simulink model "MTDC_MODEL"  (R2021a)
settings: Solver=ode1  StartTime=0.0  StopTime=3  FixedStep=2e-5  MaxStep=1e-5  RelTol=1e-5  EnableMultiTasking=on
InitFcn:
  | tau_iac=ts_G_iac/4;                                         %Current loop speed
  | wAC=1/tau_iac;                                              %Frequency
  | L1AC=wAC/s;                                                 %Open loop IMC (L) transfer function to obtain a first order after closing the loop
  | Kp_AC=wAC*(Lg_1+La_1/2);                                    %Proportional constant of the controller
  | Ki_AC=wAC*(Rg_1+Ra_1/2);                                    %Integral constant of the controller
  | C_IMC_AC=(Kp_AC*s+Ki_AC)/s;                                 %IMC designed PI controller transfer function
  | TAC=minreal((C_IMC_AC)*G_iac/(1+(C_IMC_AC)*G_iac));         %Closed loop transfer function
  | 
  | tau_Pac=ts_G_P/4;
  | D = TAC*U_ll1;
  | [C_pi,info] = pidtune(D,'PI',1/tau_Pac);
  | Ki_P = C_pi.Ki;
  | 
  | tau_Qac=ts_G_Q/4;
  | [C_piq,info] = pidtune(D,'PI',1/tau_Qac);
  | Ki_Q = C_piq.Ki;
  | 
  | 
  | tau_isum=ts_G_isum/4;                                        %Current loop speed
  | wsum=1/tau_isum;                                             %Frequency
  | L1AC=wsum/s;                                                 %Open loop IMC (L) transfer function to obtain a first order after closing the loop
  | Kp_sum=wsum*(2*La_1);                                        %Proportional constant of the controller
  | Ki_sum=wsum*(2*Ra_1);                                        %Integral constant of the controller
  | C_IMC_sum=(Kp_sum*s+Ki_sum)/s;                               %IMC designed PI controller transfer function
  | 
  | Kp_sum_PR = wc*(2*La_1);
  | Ki_sum_PR = wc*(2*Ra_1);
  | PR = (Kp_sum_PR*s^2 + 2*wc*(Kp_sum_PR+Ki_sum_PR)*s +Kp_sum_PR*w0^2)/(s^2+2*wc*s+w0^2);
  | 
  | 
  | %Energy reference for a converter arm (sum of all the submodule energies)
  | ArmEnergyRef=1/2*Carm*ArmVoltageRef^2;                      %Energy reference for a converter leg
  | LegEnergy=ArmEnergyRef*2;                                   %References for the controllers (DC side)
  | TotalEnergyRef=ArmEnergyRef*6;                              %Reference of the total energy of the converter
  | EnergyDiffabRef=0;                                          %Reference for the energy difference between legs a and b
  | EnergyDiffacRef=0;                                          %Reference for the energy difference between legs b and c
  | 
  | %References for the controllers (AC side)
  | EnergyDiffUpLowRefa=0;                                      %Reference for the energy difference upper and lower arms of phase a
  | EnergyDiffUpLowRefb=0;                                      %Reference for the energy difference upper and lower arms of phase b
  | EnergyDiffUpLowRefc=0;                                      %Reference for the energy difference upper and lower arms of phase c
  |                                                             %Controller design
  | Kpenergy=50;                                                %Proportional gain
  | Kienergy=20;                                                %Integral gain
  | 
  | Kpenergyt=50;                                               %Proportional gain
  | Kienergyt=20;                                               %Integral gain
  | 
  | Q=3;
  | wn=50*2*pi;                                                 %Frequency to eliminate 50 Hz
  | N_50 = tf([1 0 wn^2],[1 2*wn/Q wn^2]);                       %Notch filter 1 design
  | wn=100*2*pi;                                                %Frequency to eliminate 100 Hz
  | N_100 = tf([1 0 wn^2],[1 2*wn/Q wn^2]);                      %Notch filter 2 design
  | Notch=N_50*N_100;                                            %Combination of both notch filters
  | 
  | Ibasedc1= 1000e6/640e3;                 %Nominal current peak DC
  | IsaturationinnerDC1=1.1*Ibasedc1/3;  %Saturation of the DC inner current
  | IsaturationinnerAC1=0.45*Ibasedc1/3; %0.45  %Saturation of the inner current (why edu used 10% - FYI I changed it to 45%)
  | 
  | 
  | ... (+30 lines)
values from neighbouring files (symbols this model uses):
  ArmVoltageRef = 640e3    (= 640000)    [MMC_PARAMETERS.m]
  Cap = 9.5e-3    (= 0.0095)    [MMC_PARAMETERS.m]
  Carm = Cap/N    (= 2.375e-05)    [MMC_PARAMETERS.m]
  f_grid = 50    [MMC_PARAMETERS.m]
  La_1 = 0.15*Zbase_1/2/pi/50    (= 0.0488923985178)    [MMC_PARAMETERS.m]
  Lg_1 = 0.18*Zbase_1/2/pi/50    (= 0.0586708782214)    [MMC_PARAMETERS.m]
  N = 400    [MMC_PARAMETERS.m]
  Ra_1 = 0.01*Zbase_1    (= 1.024)    [MMC_PARAMETERS.m]
  Rg_1 = 0.005*Zbase_1    (= 0.512)    [MMC_PARAMETERS.m]
  S_1 = 1000e6    (= 1000000000)    [MMC_PARAMETERS.m]
  U_ll1 = 320e3    (= 320000)    [MMC_PARAMETERS.m]
  Vdc = 640e3    (= 640000)    [MMC_PARAMETERS.m]
  Vpeak_d1 = U_pnpeak1    [MMC_PARAMETERS.m]
  w0 = 2*pi*50    (= 314.159265359)    [MMC_PARAMETERS.m]
undefined symbols (not defined in the file or in its folder): Kp_Pac, lenght
libraries: spsSeriesRLCBranchLib x80, spsCurrentMeasurementLib x64, spsControlledVoltageSourceLib x36, pid_lib x32, spsVoltageMeasurementLib x32, spsControlledCurrentSourceLib x24, spsParallelRLCBranchLib x20, spsGroundLib x10, powerlib_extras x4, spsDCVoltageSourceLib x4, spspowerguiLib x1
(part 7 of 9)

== system MTDC_MODEL/GRID4+MMC4/Equivalent arm lower-a2 ==
  note: Power_lb
  vlb : Inport
  Controlled Current Source : spsControlledCurrentSourceLib/Controlled Current Source  Initialize=on  Source_Type=AC  Amplitude=0  Phase=0  Frequency=0  Measurements=None
  Controlled Voltage Source7 : spsControlledVoltageSourceLib/Controlled Voltage Source  Initialize=on  Source_Type=AC  Amplitude=Vdc/2  Phase=0  Frequency=0  Measurements=None
  Current Measurement4 : spsCurrentMeasurementLib/Current Measurement  PhasorSimulation=off  OutputType=Complex  PSBequivalent=0
  Divide1 : Product  Inputs=**
  Divide2 : Product  Inputs=*/
  Filtered Lower arm B instananeous power1 : Scope
  Gain : Gain  Gain=1e6
  Lower arm B instananeous power : Scope
  Series RLC Branch2 : spsSeriesRLCBranchLib/Series RLC Branch  LConnTagsString=__new0  RConnTagsString=__new0  BranchType=C  Resistance=Ra_1  Inductance=La_1  SetiL0=on  InitialCurrent=0  Capacitance=Cap/N  Setx0=on  InitialVoltage=640e3  Measurements=None
  Transfer Fcn : TransferFcn  Denominator=[1 1]
  Voltage Measurement : spsVoltageMeasurementLib/Voltage Measurement  PhasorSimulation=off  OutputType=Complex  PSBequivalent=0
  Conn1 : PMIOPort  Side=Right
  Conn2 : PMIOPort  Port=2  Side=Left
  v_sum_lb : Outport
  wires:
  Gain/1 -> Filtered Lower arm B instananeous power1/1
  Transfer Fcn/1 -> Gain/1
  Current Measurement4/1 -> Divide1/2  "ilb"
  Divide1/1 -> Divide2/1, Transfer Fcn/1, Lower arm B instananeous power/1
  Divide2/1 -> Controlled Current Source/1
  Voltage Measurement/1 -> Divide2/2, v_sum_lb/1
  vlb/1 -> Controlled Voltage Source7/1, Divide1/1  "vlb"
  connections:
  Conn2/RConn1 -- Current Measurement4/RConn1
  Current Measurement4/LConn1 -- Controlled Voltage Source7/LConn1
  Voltage Measurement/LConn2 -- Series RLC Branch2/RConn1 -- Controlled Current Source/LConn1
  Controlled Current Source/RConn1 -- Series RLC Branch2/LConn1 -- Voltage Measurement/LConn1
  Controlled Voltage Source7/RConn1 -- Conn1/RConn1

== system MTDC_MODEL/GRID4+MMC4/Equivalent arm lower-a3 ==
  note: Power_lc
  vlc : Inport
  Controlled Current Source : spsControlledCurrentSourceLib/Controlled Current Source  Initialize=on  Source_Type=AC  Amplitude=0  Phase=0  Frequency=0  Measurements=None
  Controlled Voltage Source7 : spsControlledVoltageSourceLib/Controlled Voltage Source  Initialize=on  Source_Type=AC  Amplitude=Vdc/2  Phase=0  Frequency=0  Measurements=None
  Current Measurement4 : spsCurrentMeasurementLib/Current Measurement  PhasorSimulation=off  OutputType=Complex  PSBequivalent=0
  Divide1 : Product  Inputs=**
  Divide2 : Product  Inputs=*/
  Filtered Lower arm A instananeous power1 : Scope
  Gain : Gain  Gain=1e6
  Lower arm A instananeous power : Scope
  Series RLC Branch2 : spsSeriesRLCBranchLib/Series RLC Branch  LConnTagsString=__new0  RConnTagsString=__new0  BranchType=C  Resistance=Ra_1  Inductance=La_1  SetiL0=on  InitialCurrent=0  Capacitance=Cap/N  Setx0=on  InitialVoltage=640e3  Measurements=None
  Transfer Fcn : TransferFcn  Denominator=[1 1]
  Voltage Measurement : spsVoltageMeasurementLib/Voltage Measurement  PhasorSimulation=off  OutputType=Complex  PSBequivalent=0
  Conn1 : PMIOPort  Side=Right
  Conn2 : PMIOPort  Port=2  Side=Left
  v_sum_lc : Outport
  wires:
  vlc/1 -> Divide1/1, Controlled Voltage Source7/1  "vla"
  Voltage Measurement/1 -> v_sum_lc/1, Divide2/2
  Divide2/1 -> Controlled Current Source/1
  Divide1/1 -> Lower arm A instananeous power/1, Transfer Fcn/1, Divide2/1
  Current Measurement4/1 -> Divide1/2  "ila"
  Transfer Fcn/1 -> Gain/1
  Gain/1 -> Filtered Lower arm A instananeous power1/1
  connections:
  Controlled Voltage Source7/RConn1 -- Conn1/RConn1
  Voltage Measurement/LConn1 -- Series RLC Branch2/LConn1 -- Controlled Current Source/RConn1
  Controlled Current Source/LConn1 -- Series RLC Branch2/RConn1 -- Voltage Measurement/LConn2
  Current Measurement4/LConn1 -- Controlled Voltage Source7/LConn1
  Conn2/RConn1 -- Current Measurement4/RConn1

== system MTDC_MODEL/GRID4+MMC4/Equivalent arm upper-a ==
  note: Power_ua
  vua : Inport
  Controlled Current Source : spsControlledCurrentSourceLib/Controlled Current Source  Initialize=on  Source_Type=AC  Amplitude=0  Phase=0  Frequency=0  Measurements=None
  Controlled Voltage Source7 : spsControlledVoltageSourceLib/Controlled Voltage Source  Initialize=on  Source_Type=AC  Amplitude=Vdc/2  Phase=0  Frequency=0  Measurements=None
  Current Measurement4 : spsCurrentMeasurementLib/Current Measurement  PhasorSimulation=off  OutputType=Complex  PSBequivalent=0
  Divide1 : Product  Inputs=**
  Divide2 : Product  Inputs=*/
  Filtered Upper arm A instananeous power1 : Scope
  Gain : Gain  Gain=1e6
  Series RLC Branch2 : spsSeriesRLCBranchLib/Series RLC Branch  LConnTagsString=__new0  RConnTagsString=__new0  BranchType=C  Resistance=Ra_1  Inductance=La_1  SetiL0=on  InitialCurrent=0  Capacitance=Cap/N  Setx0=on  InitialVoltage=640e3  Measurements=None
  Transfer Fcn : TransferFcn  Denominator=[1 1]
  Upper arm A instananeous power : Scope
  Voltage Measurement : spsVoltageMeasurementLib/Voltage Measurement  PhasorSimulation=off  OutputType=Complex  PSBequivalent=0
  Conn1 : PMIOPort  Side=Right
  Conn2 : PMIOPort  Port=2  Side=Left
  v_sum_ua : Outport
  wires:
  Gain/1 -> Filtered Upper arm A instananeous power1/1
  Transfer Fcn/1 -> Gain/1
  Current Measurement4/1 -> Divide1/2  "iua"
  Divide1/1 -> Divide2/1, Transfer Fcn/1, Upper arm A instananeous power/1
  Divide2/1 -> Controlled Current Source/1
  Voltage Measurement/1 -> Divide2/2, v_sum_ua/1
  vua/1 -> Controlled Voltage Source7/1, Divide1/1  "vua"
  connections:
  Conn2/RConn1 -- Current Measurement4/RConn1
  Current Measurement4/LConn1 -- Controlled Voltage Source7/LConn1
  Voltage Measurement/LConn2 -- Series RLC Branch2/RConn1 -- Controlled Current Source/LConn1
  Controlled Current Source/RConn1 -- Series RLC Branch2/LConn1 -- Voltage Measurement/LConn1
  Controlled Voltage Source7/RConn1 -- Conn1/RConn1

== system MTDC_MODEL/GRID4+MMC4/Equivalent arm upper-b ==
  note: Power_ub
  vub : Inport
  Controlled Current Source : spsControlledCurrentSourceLib/Controlled Current Source  Initialize=on  Source_Type=AC  Amplitude=0  Phase=0  Frequency=0  Measurements=None
  Controlled Voltage Source7 : spsControlledVoltageSourceLib/Controlled Voltage Source  Initialize=on  Source_Type=AC  Amplitude=Vdc/2  Phase=0  Frequency=0  Measurements=None
  Current Measurement4 : spsCurrentMeasurementLib/Current Measurement  PhasorSimulation=off  OutputType=Complex  PSBequivalent=0
  Divide1 : Product  Inputs=**
  Divide2 : Product  Inputs=*/
  Filtered Upper arm A instananeous power1 : Scope
  Gain : Gain  Gain=1e6
  Series RLC Branch2 : spsSeriesRLCBranchLib/Series RLC Branch  LConnTagsString=__new0  RConnTagsString=__new0  BranchType=C  Resistance=Ra_1  Inductance=La_1  SetiL0=on  InitialCurrent=0  Capacitance=Cap/N  Setx0=on  InitialVoltage=640e3  Measurements=None
  Transfer Fcn : TransferFcn  Denominator=[1 1]
  Upper arm A instananeous power : Scope
  Voltage Measurement : spsVoltageMeasurementLib/Voltage Measurement  PhasorSimulation=off  OutputType=Complex  PSBequivalent=0
  Conn1 : PMIOPort  Side=Right
  Conn2 : PMIOPort  Port=2  Side=Left
  v_sum_ub : Outport
  wires:
  Gain/1 -> Filtered Upper arm A instananeous power1/1
  Transfer Fcn/1 -> Gain/1
  Current Measurement4/1 -> Divide1/2  "iub"
  Divide1/1 -> Divide2/1, Transfer Fcn/1, Upper arm A instananeous power/1
  Divide2/1 -> Controlled Current Source/1
  Voltage Measurement/1 -> Divide2/2, v_sum_ub/1
  vub/1 -> Controlled Voltage Source7/1, Divide1/1  "vub"
  connections:
  Conn2/RConn1 -- Current Measurement4/RConn1
  Current Measurement4/LConn1 -- Controlled Voltage Source7/LConn1
  Voltage Measurement/LConn2 -- Series RLC Branch2/RConn1 -- Controlled Current Source/LConn1
  Controlled Current Source/RConn1 -- Series RLC Branch2/LConn1 -- Voltage Measurement/LConn1
  Controlled Voltage Source7/RConn1 -- Conn1/RConn1

== system MTDC_MODEL/GRID4+MMC4/Equivalent arm upper-c ==
  note: Power_uc
  vuc : Inport
  Controlled Current Source : spsControlledCurrentSourceLib/Controlled Current Source  Initialize=on  Source_Type=AC  Amplitude=0  Phase=0  Frequency=0  Measurements=None
  Controlled Voltage Source7 : spsControlledVoltageSourceLib/Controlled Voltage Source  Initialize=on  Source_Type=AC  Amplitude=Vdc/2  Phase=0  Frequency=0  Measurements=None
  Current Measurement4 : spsCurrentMeasurementLib/Current Measurement  PhasorSimulation=off  OutputType=Complex  PSBequivalent=0
  Divide1 : Product  Inputs=**
  Divide2 : Product  Inputs=*/
  Filtered Upper arm A instananeous power1 : Scope
  Gain : Gain  Gain=1e6
  Series RLC Branch2 : spsSeriesRLCBranchLib/Series RLC Branch  LConnTagsString=__new0  RConnTagsString=__new0  BranchType=C  Resistance=Ra_1  Inductance=La_1  SetiL0=on  InitialCurrent=0  Capacitance=Cap/N  Setx0=on  InitialVoltage=640e3  Measurements=None
  Transfer Fcn : TransferFcn  Denominator=[1 1]
  Upper arm A instananeous power : Scope
  Voltage Measurement : spsVoltageMeasurementLib/Voltage Measurement  PhasorSimulation=off  OutputType=Complex  PSBequivalent=0
  Conn1 : PMIOPort  Side=Right
  Conn2 : PMIOPort  Port=2  Side=Left
  v_sum_uc : Outport
  wires:
  Gain/1 -> Filtered Upper arm A instananeous power1/1
  Transfer Fcn/1 -> Gain/1
  Current Measurement4/1 -> Divide1/2  "iuc"
  Divide1/1 -> Divide2/1, Transfer Fcn/1, Upper arm A instananeous power/1
  Divide2/1 -> Controlled Current Source/1
  Voltage Measurement/1 -> Divide2/2, v_sum_uc/1
  vuc/1 -> Controlled Voltage Source7/1, Divide1/1  "vuc"
  connections:
  Conn2/RConn1 -- Current Measurement4/RConn1
  Current Measurement4/LConn1 -- Controlled Voltage Source7/LConn1
  Voltage Measurement/LConn2 -- Series RLC Branch2/RConn1 -- Controlled Current Source/LConn1
  Controlled Current Source/RConn1 -- Series RLC Branch2/LConn1 -- Voltage Measurement/LConn1
  Controlled Voltage Source7/RConn1 -- Conn1/RConn1

== system MTDC_MODEL/GRID4+MMC4/Feedforward calculation ==
  vzabc : Inport
  isabc : Inport  Port=2
  Demux1 : Demux  Outputs=3
  First order filter1 : Subsystem
  Mux2 : Mux  Inputs=2
  PI10 : TransferFcn  Numerator=[Notch.num{1}]  Denominator=[Notch.den{1}]
  PI9 : TransferFcn  Numerator=[Notch.num{1}]  Denominator=[Notch.den{1}]
  Product5 : Product
  Scope3 : Scope
  Sum15 : Sum  Inputs=|+-
  Sum39 : Sum  Inputs=|+-
  Sum5 : Sum  Inputs=+++
  Pt : Outport  VectorParamsAs1DForOutWhenUnconnected=off
  Pab : Outport  Port=2  VectorParamsAs1DForOutWhenUnconnected=off
  Pac : Outport  Port=3  VectorParamsAs1DForOutWhenUnconnected=off
  wires:
  PI10/1 -> Mux2/2
  PI9/1 -> Mux2/1
  Mux2/1 -> Scope3/1
  Sum5/1 -> Pt/1
  isabc/1 -> Product5/2
  First order filter1/1(Out1) -> Demux1/1
  Product5/1 -> First order filter1/1(In1)
  Sum39/1 -> PI10/1, Pac/1  "Pb-Pc"
  Sum15/1 -> PI9/1, Pab/1  "Pa-Pb"
  vzabc/1 -> Product5/1
  Demux1/1 -> Sum5/1, Sum39/1, Sum15/1
  Demux1/2 -> Sum5/2, Sum15/2
  Demux1/3 -> Sum5/3, Sum39/2

== system MTDC_MODEL/GRID4+MMC4/Grid3 ==
  Constant : Constant
  Constant1 : Constant  Value=f_grid
  Constant{2,5..7,20} (5 alike) : Constant  Value=0
  Constant21 : Constant  Value=-2*pi/3
  Constant22 : Constant  Value=2*pi/3
  Constant8 : Constant  Value=2*pi/3
  Constant9 : Constant  Value=-2*pi/3
  Gain1 : Gain  Gain=2*pi
  Gain{2..3,6,8} (4 alike) : Gain  Gain=Vpeak_d1
  Gain4 : Gain  Gain=0
  Gain5 : Gain  Gain=0
  Gain7 : Gain  Gain=0
  Integrator{1..3,8..10} (6 alike) : Integrator
  Sum{1..12} (12 alike) : Sum  Inputs=|++
  Trigonometric Function{1..3,6..8} (6 alike) : Trigonometry  Operator=cos
  vza : Outport
  vzb : Outport  Port=2
  vzc : Outport  Port=3
  thetareal : Outport  Port=4
  vpos : Outport  Port=5
  wires:
  Gain6/1 -> vpos/1
  Constant/1 -> Gain6/1
  Sum8/1 -> Trigonometric Function8/1
  Integrator9/1 -> Sum7/1
  Trigonometric Function6/1 -> Gain8/1
  Constant20/1 -> Sum9/2
  Sum7/1 -> Trigonometric Function7/1
  Integrator8/1 -> Sum9/1
  Constant21/1 -> Sum7/2
  Integrator10/1 -> Sum8/1
  Constant22/1 -> Sum8/2
  Sum9/1 -> Trigonometric Function6/1, thetareal/1
  Constant1/1 -> Gain1/1
  Trigonometric Function8/1 -> Gain3/1
  Trigonometric Function7/1 -> Gain2/1
  Gain8/1 -> Sum4/1
  Gain2/1 -> Sum5/1
  Gain3/1 -> Sum6/1
  Sum2/1 -> Trigonometric Function3/1
  Integrator3/1 -> Sum1/1
  Trigonometric Function1/1 -> Gain7/1
  Constant7/1 -> Sum3/2
  Sum1/1 -> Trigonometric Function2/1
  Gain1/1 -> Integrator3/1, Integrator1/1, Integrator2/1, Integrator10/1, Integrator8/1, Integrator9/1
  Integrator2/1 -> Sum3/1
  Constant8/1 -> Sum1/2
  Integrator1/1 -> Sum2/1
  Constant9/1 -> Sum2/2
  Sum3/1 -> Trigonometric Function1/1
  Trigonometric Function3/1 -> Gain5/1
  Trigonometric Function2/1 -> Gain4/1
  Gain7/1 -> Sum4/2
  Gain4/1 -> Sum5/2
  Gain5/1 -> Sum6/2
  Sum4/1 -> Sum10/1
  Sum5/1 -> Sum11/1
  Sum6/1 -> Sum12/1
  Constant2/1 -> Sum10/2
  Constant5/1 -> Sum11/2
  Constant6/1 -> Sum12/2
  Sum10/1 -> vza/1
  Sum11/1 -> vzb/1
  Sum12/1 -> vzc/1

== system MTDC_MODEL/GRID4+MMC4/Isum_AC_Ref_Cal ==
  note: positive sequence
  note: negative sequence
  Pdiff_arm_a_Ref : Inport
  Pdiff_arm_b_Ref : Inport  Port=2
  Pdiff_arm_c_Ref : Inport  Port=3
  Clarke : Inport  Port=4
  v_g_pos : Inport  Port=5
  theta : Inport  Port=6
  Constant5 : Constant  Value=0
  Constant7 : Constant  Value=0
  "DIFFERENT_REF_CALC_METHODS " : Subsystem
  Demux2 : Demux
  Demux3 : Demux  Outputs=3
  Display : Display
  Gain1 : Gain  Gain=1/S_1
  Gain10 : Gain  Gain=-1
  Gain11 : Gain  Gain=sqrt(2)
  Gain19 : Gain  Gain=S_1/(U_ll1)
  Gain2 : Gain  Gain=1/S_1
  Gain3 : Gain  Gain=1/S_1
  Matrix Multiply{,1..2,6} (4 alike) : Product  Multiplication=Matrix(*)
  Mux28 : Mux  Inputs=2
  Mux57 : Mux  Inputs=3
  Mux6 : Mux
  Mux8 : Mux  Inputs=2
  Mux9 : Mux  Inputs=2
  Rotation4 : Subsystem
  Scope4 : Scope
  Sum7 : Sum  Inputs=+|+
  i_albe_AC : Outport  VectorParamsAs1DForOutWhenUnconnected=off
  wires:
  v_g_pos/1 -> "DIFFERENT_REF_CALC_METHODS "/1(v_g_pos)
  Mux9/1 -> Matrix Multiply6/2
  Mux8/1 -> Matrix Multiply/2
  theta/1 -> Rotation4/1(angle)
  Rotation4/1(iR) -> [iR]
  Rotation4/2(R) -> [R]
  Demux2/4 -> Mux9/2
  Demux2/1 -> Mux8/1
  Sum7/1 -> Mux28/1
  Demux2/2 -> Mux8/2
  Demux2/3 -> Mux9/1
  Matrix Multiply6/1 -> Sum7/2
  Mux28/1 -> i_albe_AC/1
  Matrix Multiply/1 -> Sum7/1
  Gain11/1 -> Demux2/1, Scope4/1
  Constant5/1 -> Mux28/2
  [iR] -> Matrix Multiply6/1
  [R] -> Matrix Multiply/1
  Gain19/1 -> Gain11/1
  Gain1/1 -> Mux57/3
  Gain2/1 -> Mux57/2
  Gain3/1 -> Mux57/1
  Clarke/1 -> Matrix Multiply1/1
  Pdiff_arm_c_Ref/1 -> Gain1/1
  Pdiff_arm_b_Ref/1 -> Gain2/1
  Pdiff_arm_a_Ref/1 -> Gain3/1
  Demux3/3 -> Mux6/3  "Isum_pos"
  Gain10/1 -> Mux6/2
  Demux3/2 -> Gain10/1  "-Isum_neg"
  Demux3/1 -> Mux6/1  "Isum_neg"
  Matrix Multiply2/1 -> Demux3/1
  Constant7/1 -> Mux6/4
  Mux6/1 -> Gain19/1
  "DIFFERENT_REF_CALC_METHODS "/1(Initial Approach) -> Matrix Multiply2/1, Display/1
  Matrix Multiply1/1 -> Matrix Multiply2/2  "P_al; P_be; P_0"
  Mux57/1 -> Matrix Multiply1/2

== system MTDC_MODEL/GRID4+MMC4/Modulation ==
  vdiffabc : Inport
  vsumabc : Inport  Port=2
  Constant12 : Constant  Value=[-1 0 0 1/2 0 0;0 -1 0 0 1/2 0 ;0 0 -1 0 0 1/2;1 0 0 1/2 0 0;0 1 0 0 1/2 0;0 0 1 0 0 1/2]  SampleTime=-1
  Demux3 : Demux  Outputs=6
  Gain1 : Gain  Gain=-1
  Matrix Multiply1 : Product  Multiplication=Matrix(*)
  Mux12 : Mux  Inputs=2
  Mux17 : Mux  Inputs=3
  Mux19 : Mux  Inputs=3
  vuabc : Outport
  vlabc : Outport  Port=2
  wires:
  Demux3/4 -> Mux19/1
  Demux3/5 -> Mux19/2
  Demux3/6 -> Mux19/3
  Demux3/1 -> Mux17/1
  Demux3/2 -> Mux17/2
  Demux3/3 -> Mux17/3
  Mux19/1 -> vlabc/1
  Mux17/1 -> vuabc/1
  vsumabc/1 -> Gain1/1
  Gain1/1 -> Mux12/2
  Matrix Multiply1/1 -> Demux3/1
  vdiffabc/1 -> Mux12/1
  Mux12/1 -> Matrix Multiply1/2
  Constant12/1 -> Matrix Multiply1/1

== system MTDC_MODEL/GRID4+MMC4/Park//nPark2 ==
  theta : Inport
  Constant1 : Constant  Value=1/2  SampleTime=0
  Constant2 : Constant  Value=1/2  SampleTime=0
  Constant3 : Constant  Value=1/2  SampleTime=0
  Constant4 : Constant  Value=2*pi/3  SampleTime=0
  Constant5 : Constant  SampleTime=0
  Constant6 : Constant  SampleTime=0
  Constant7 : Constant  SampleTime=0
  Gain7 : Gain  Gain=2/3
  Matrix Concatenate1 : Concatenate  NumInputs=3  Mode=Multidimensional array  ConcatenateDimension=2
  Matrix Concatenate2 : Concatenate  NumInputs=3  Mode=Multidimensional array  ConcatenateDimension=2
  Mux{1..6} (6 alike) : Mux  Inputs=3
  Sum1 : Sum  Inputs=|++
  Sum2 : Sum  Inputs=|+-
  Trigonometric Function : Trigonometry  Operator=cos
  Trigonometric Function1 : Trigonometry
  Trigonometric Function2 : Trigonometry  Operator=cos
  Trigonometric Function3 : Trigonometry
  Trigonometric Function4 : Trigonometry  Operator=cos
  Trigonometric Function5 : Trigonometry
  T : Outport
  "nT " : Outport  Port=2
  wires:
  Mux4/1 -> Matrix Concatenate2/3
  Constant7/1 -> Mux4/3
  Constant6/1 -> Mux4/2
  Constant5/1 -> Mux4/1
  Constant3/1 -> Mux3/3
  Constant2/1 -> Mux1/3
  Constant1/1 -> Mux2/3
  Sum2/1 -> Trigonometric Function2/1, Trigonometric Function3/1
  Sum1/1 -> Trigonometric Function4/1, Trigonometric Function5/1
  Constant4/1 -> Sum2/2, Sum1/2
  Trigonometric Function/1 -> Mux2/1, Mux5/1
  Trigonometric Function1/1 -> Mux2/2, Mux6/1
  Trigonometric Function2/1 -> Mux5/2, Mux1/1
  Trigonometric Function3/1 -> Mux6/2, Mux1/2
  Trigonometric Function4/1 -> Mux3/1, Mux5/3
  Trigonometric Function5/1 -> Mux6/3, Mux3/2
  Mux2/1 -> Matrix Concatenate1/1
  Mux1/1 -> Matrix Concatenate1/2
  Mux3/1 -> Matrix Concatenate1/3
  Matrix Concatenate1/1 -> Gain7/1
  Mux5/1 -> Matrix Concatenate2/1
  Mux6/1 -> Matrix Concatenate2/2
  theta/1 -> Sum1/1, Sum2/1, Trigonometric Function/1, Trigonometric Function1/1
  Gain7/1 -> T/1
  Matrix Concatenate2/1 -> "nT "/1

== system MTDC_MODEL/GRID4+MMC4/Power_calculation ==
  Pua : Inport
  Pla : Inport  Port=2
  Pub : Inport  Port=3
  Plb : Inport  Port=4
  Puc : Inport  Port=5
  Plc : Inport  Port=6
  Sum : Sum
  Sum1 : Sum
  Sum2 : Sum
  Sum3 : Sum  Inputs=+++
  Sum{4..8} (5 alike) : Sum  Inputs=+-
  Pab : Outport
  Pac : Outport  Port=2
  Pt : Outport  Port=3
  Pula : Outport  Port=4
  Pulb : Outport  Port=5
  Pulc : Outport  Port=6
  wires:
  Sum8/1 -> Pulc/1
  Puc/1 -> Sum8/1, Sum2/1
  Plc/1 -> Sum2/2, Sum8/2
  Plb/1 -> Sum1/2, Sum5/2
  Pub/1 -> Sum1/1, Sum5/1
  Sum5/1 -> Pulb/1
  Sum4/1 -> Pula/1
  Pua/1 -> Sum/1, Sum4/1
  Sum7/1 -> Pac/1
  Sum6/1 -> Pab/1
  Pla/1 -> Sum/2, Sum4/2
  Sum1/1 -> Sum6/2, Sum3/1
  Sum/1 -> Sum6/1, Sum7/1, Sum3/2
  Sum3/1 -> Pt/1
  Sum2/1 -> Sum7/2, Sum3/3

== system MTDC_MODEL/GRID4+MMC4/Subsystem1 ==
  Uuabc : Inport
  Iuabc : Inport  Port=2
  Ulabc : Inport  Port=3
  Ilabc : Inport  Port=4
  Demux{,2,4,6} (4 alike) : Demux  Outputs=3
  Product{,1..5} (6 alike) : Product
  Pua : Outport
  Pub : Outport  Port=2
  Puc : Outport  Port=3
  Pla : Outport  Port=4
  Plb : Outport  Port=5
  Plc : Outport  Port=6
  wires:
  Iuabc/1 -> Demux2/1
  Product2/1 -> Puc/1
  Product4/1 -> Plb/1
  Product3/1 -> Pla/1
  Product1/1 -> Pub/1
  Product/1 -> Pua/1
  Demux/2 -> Product1/1
  Demux/3 -> Product2/1
  Ilabc/1 -> Demux6/1
  Demux4/1 -> Product3/1
  Demux4/2 -> Product4/1
  Demux4/3 -> Product5/1
  Product5/1 -> Plc/1
  Demux/1 -> Product/1
  Demux6/1 -> Product3/2
  Demux2/3 -> Product2/2
  Uuabc/1 -> Demux/1
  Demux2/1 -> Product/2
  Ulabc/1 -> Demux4/1
  Demux6/3 -> Product5/2
  Demux2/2 -> Product1/2
  Demux6/2 -> Product4/2

== system MTDC_MODEL/GRID4+MMC4/Voltage calculation ==
  vus_a : Inport
  vus_b : Inport  Port=2
  vus_c : Inport  Port=3
  vls_a : Inport  Port=4
  vls_b : Inport  Port=5
  vls_c : Inport  Port=6
  Mux11 : Mux  Inputs=3
  Sum : Sum  Inputs=|++
  Sum10 : Sum  Inputs=|++
  Sum11 : Sum  Inputs=+-|
  Sum12 : Sum  Inputs=+++
  Sum2 : Sum  Inputs=+-|
  Sum9 : Sum  Inputs=|++
  v_total_abc : Outport
  V_diff_ab : Outport  Port=2
  V_diff_ac : Outport  Port=3
  V_t_MMC : Outport  Port=4
  wires:
  vls_a/1 -> Sum/2
  Sum12/1 -> V_t_MMC/1  "V_t_MMC"
  vus_b/1 -> Sum9/1
  Sum2/1 -> V_diff_ac/1  "V_diff_ac"
  vls_b/1 -> Sum9/2
  Sum9/1 -> Sum12/2, Mux11/2, Sum11/2  "v_total_b"
  Sum10/1 -> Sum12/3, Mux11/3, Sum2/2  "v_total_c"
  vus_a/1 -> Sum/1
  Sum11/1 -> V_diff_ab/1  "V_diff_ab"
  Mux11/1 -> v_total_abc/1
  vls_c/1 -> Sum10/2
  Sum/1 -> Sum2/1, Sum12/1, Mux11/1, Sum11/1  "v_total_a"
  vus_c/1 -> Sum10/1

== system MTDC_MODEL/GRID4+MMC4/Voltage calculation1 ==
  vus_a : Inport
  vus_b : Inport  Port=2
  vus_c : Inport  Port=3
  vls_a : Inport  Port=4
  vls_b : Inport  Port=5
  vls_c : Inport  Port=6
  Sum : Sum  Inputs=|+-
  Sum10 : Sum  Inputs=|+-
  Sum9 : Sum  Inputs=|+-
  v_total_a : Outport
  v_total_b : Outport  Port=2
  v_total_c : Outport  Port=3
  wires:
  vus_c/1 -> Sum10/1
  Sum/1 -> v_total_a/1  "v_total_a"
  vls_c/1 -> Sum10/2
  vus_a/1 -> Sum/1
  Sum10/1 -> v_total_c/1  "v_total_c"
  Sum9/1 -> v_total_b/1  "v_total_b"
  vls_b/1 -> Sum9/2
  vus_b/1 -> Sum9/1
  vls_a/1 -> Sum/2

== system MTDC_MODEL/GRID4+MMC4/vsum Calculation ==
  Inner_current_refs : Inport
  i_uabc : Inport  Port=2
  i_labc : Inport  Port=3
  irefabcDC : Inport  Port=4
  Constant : Constant  Value=640e3
  Constant15 : Constant  Value="[1  0 0 1 0 0;0 1 0 0 1 0 ;0 0 1 0 0 1]"  SampleTime=-1
  Demux1 : Demux  Outputs=3
  Demux3 : Demux  Outputs=3
  Demux7 : Demux  Outputs=3
  Gain1 : Gain  Gain=1/2
  Matrix Multiply{2,10,13,18} (4 alike) : Product  Multiplication=Matrix(*)
  Memory : Memory
  Memory1 : Memory
  Memory2 : Memory  InitialCondition=-Vdc
  Mux13 : Mux  Inputs=3
  Mux18 : Mux  Inputs=2
  PR Controller1 : Subsystem
  PR Controller2 : Subsystem
  PR Controller3 : Subsystem
  SMC : Subsystem
  Sum{3,5..6,11} (4 alike) : Sum  Inputs=|+-
  Sum13 : Sum  Inputs=++|
  vsumqd0 : Scope  NumInputPorts=3
  vsumqd1 : Scope  NumInputPorts=3
  vsumabc : Outport  VectorParamsAs1DForOutWhenUnconnected=off
  wires:
  Memory2/1 -> vsumqd1/1, Mux13/3
  Demux1/2 -> vsumqd0/2
  Demux1/1 -> vsumqd0/1
  Demux1/3 -> vsumqd0/3, vsumqd1/2
  SMC/1(Out1) -> Demux1/1
  Inner_current_refs/1 -> Sum13/1
  Memory1/1 -> Mux13/2
  Memory/1 -> Mux13/1
  Matrix Multiply10/1 -> vsumabc/1
  i_labc/1 -> Mux18/2
  i_uabc/1 -> Mux18/1
  [Clarke] -> Matrix Multiply2/1
  [Clarke] -> Matrix Multiply18/1
  [nC] -> Matrix Multiply10/1
  Matrix Multiply2/1 -> Demux3/1
  Demux7/1 -> Sum5/1
  Matrix Multiply13/1 -> Gain1/1
  Constant15/1 -> Matrix Multiply13/1
  Mux18/1 -> Matrix Multiply13/2
  irefabcDC/1 -> Matrix Multiply18/2
  Constant/1 -> Sum11/2
  Matrix Multiply18/1 -> Sum13/2
  Sum11/1 -> Memory2/1
  PR Controller3/1(v) -> Sum11/1
  Demux3/2 -> Sum3/2
  PR Controller2/1(v) -> Memory1/1
  Sum3/1 -> SMC/2(S_beta), PR Controller2/1(e)
  Sum6/1 -> SMC/3(S_0), PR Controller3/1(e)
  Sum5/1 -> SMC/1(S_alfa), PR Controller1/1(e)
  PR Controller1/1(v) -> Memory/1
  Demux3/3 -> Sum6/2
  Demux7/2 -> Sum3/1
  Demux7/3 -> Sum6/1
  Demux3/1 -> Sum5/2
  Sum13/1 -> Demux7/1, SMC/4(i_ref)
  Gain1/1 -> Matrix Multiply2/2
  Mux13/1 -> Matrix Multiply10/2

== system MTDC_MODEL/GRID1+MMC1/DC References/Sat3 ==
  In1 : Inport
  Demux4 : Demux  Outputs=3
  Mux5 : Mux  Inputs=3
  Saturation1 : Saturate  UpperLimit=IsaturationinnerDC1  LowerLimit=-IsaturationinnerDC1
  Saturation4 : Saturate  UpperLimit=IsaturationinnerDC1  LowerLimit=-IsaturationinnerDC1
  Saturation5 : Saturate  UpperLimit=IsaturationinnerDC1  LowerLimit=-IsaturationinnerDC1
  Out1 : Outport  VectorParamsAs1DForOutWhenUnconnected=off
  wires:
  Saturation5/1 -> Mux5/3
  Saturation4/1 -> Mux5/2
  Saturation1/1 -> Mux5/1
  Demux4/3 -> Saturation5/1
  Demux4/2 -> Saturation4/1
  Demux4/1 -> Saturation1/1
  Mux5/1 -> Out1/1
  In1/1 -> Demux4/1

== system MTDC_MODEL/GRID1+MMC1/Energy Calculation1/AC Power Reference ==
  Ediff_arm_a : Inport
  Ediff_arm_b : Inport  Port=2
  Ediff_arm_c : Inport  Port=3
  Constant1 : Constant  Value=EnergyDiffUpLowRefb
  Constant2 : Constant  Value=EnergyDiffUpLowRefc
  Constant21 : Constant  Value=EnergyDiffUpLowRefa
  Mux : Mux  Inputs=3
  PI1 : TransferFcn  Numerator=[Notch.num{1}]  Denominator=[Notch.den{1}]
  PI2 : TransferFcn  Numerator=[Notch.num{1}]  Denominator=[Notch.den{1}]
  PI3 : Subsystem
  PI4 : Subsystem
  PI5 : Subsystem
  PI6 : TransferFcn  Numerator=[Notch.num{1}]  Denominator=[Notch.den{1}]
  Product : Product
  Scope : Scope
  Step : Step  Time=2.1  Before=1  SampleTime=0
  Sum20 : Sum  Inputs=|+-
  Sum21 : Sum  Inputs=|+-
  Sum25 : Sum  Inputs=|+-
  Pdiff_arm_a_Ref : Outport  VectorParamsAs1DForOutWhenUnconnected=off
  Pdiff_arm_b_Ref : Outport  Port=2  VectorParamsAs1DForOutWhenUnconnected=off
  Pdiff_arm_c_Ref : Outport  Port=3  VectorParamsAs1DForOutWhenUnconnected=off
  wires:
  Constant21/1 -> Sum20/1
  Sum25/1 -> PI5/1(e)
  Constant1/1 -> Sum21/1
  Constant2/1 -> Sum25/1
  Sum21/1 -> PI4/1(e)
  Ediff_arm_c/1 -> Mux/3, Sum25/2
  Ediff_arm_a/1 -> Mux/1, Sum20/2
  PI6/1 -> Pdiff_arm_c_Ref/1
  PI5/1(u) -> PI6/1
  PI1/1 -> Pdiff_arm_a_Ref/1
  Sum20/1 -> Product/1
  Ediff_arm_b/1 -> Mux/2, Sum21/2
  PI2/1 -> Pdiff_arm_b_Ref/1
  PI3/1(u) -> PI1/1
  PI4/1(u) -> PI2/1
  Product/1 -> PI3/1(e)
  Step/1 -> Product/2
  Mux/1 -> Scope/1

== system MTDC_MODEL/GRID1+MMC1/Energy Calculation1/DC Energy PIs ==
  EnergyTotal : Inport
  Energydiffab : Inport  Port=2
  Energydiffac : Inport  Port=3
  ACpowerFFd : Inport  Port=4
  DiffabABpowerFFd : Inport  Port=5
  DiffacACpowerFFd : Inport  Port=6
  Constant20 : Constant  Value=TotalEnergyRef
  Constant23 : Constant  Value=EnergyDiffabRef
  Constant29 : Constant  Value=EnergyDiffacRef
  Gain1 : Gain
  Gain43 : Gain
  Gain6 : Gain
  Mux : Mux  Inputs=2
  PI1 : TransferFcn  Numerator=[Notch.num{1}]  Denominator=[Notch.den{1}]
  PI10 : TransferFcn  Numerator=[Notch.num{1}]  Denominator=[Notch.den{1}]
  PI2 : TransferFcn  Numerator=[Notch.num{1}]  Denominator=[Notch.den{1}]
  PI3 : TransferFcn  Numerator=[Kpenergyt Kienergyt]  Denominator=[1 0 ]
  PI4 : TransferFcn  Numerator=[Kpenergyt Kienergyt]  Denominator=[1 0 ]
  PI5 : TransferFcn  Numerator=[Kpenergyt Kienergyt]  Denominator=[1 0 ]
  Scope : Scope
  Scope1 : Scope
  Sum10 : Sum  Inputs=|++
  Sum17 : Sum  Inputs=|++
  Sum20 : Sum  Inputs=|+-
  Sum21 : Sum  Inputs=|+-
  Sum25 : Sum  Inputs=|+-
  Sum27 : Sum  Inputs=|++
  TotalPowerRef : Outport  VectorParamsAs1DForOutWhenUnconnected=off
  DiffabPowerRef : Outport  Port=2  VectorParamsAs1DForOutWhenUnconnected=off
  DiffacPowerRef : Outport  Port=3  VectorParamsAs1DForOutWhenUnconnected=off
  wires:
  Constant20/1 -> Sum20/1
  Sum20/1 -> PI3/1
  Sum25/1 -> PI5/1
  Constant23/1 -> Sum21/1
  Constant29/1 -> Sum25/1
  Sum21/1 -> PI4/1
  PI5/1 -> Gain6/1
  Energydiffab/1 -> Mux/1, Sum21/2
  Energydiffac/1 -> Mux/2, Sum25/2
  EnergyTotal/1 -> Scope1/1, Sum20/2
  PI3/1 -> Gain1/1
  PI4/1 -> Gain43/1
  PI2/1 -> DiffabPowerRef/1
  PI10/1 -> DiffacPowerRef/1
  Gain43/1 -> Sum10/1
  Sum17/1 -> PI10/1
  Gain6/1 -> Sum17/1
  Sum10/1 -> PI2/1
  ACpowerFFd/1 -> Sum27/2
  Gain1/1 -> Sum27/1
  PI1/1 -> TotalPowerRef/1
  Sum27/1 -> PI1/1
  DiffacACpowerFFd/1 -> Sum17/2
  DiffabABpowerFFd/1 -> Sum10/2
  Mux/1 -> Scope/1

== system MTDC_MODEL/GRID1+MMC1/Feedforward calculation/First order filter1 ==
  In1 : Inport
  Demux11 : Demux  Outputs=3
  Mux23 : Mux  Inputs=3
  R1 : TransferFcn  Numerator=1  Denominator=[tau_isum 1]
  R2 : TransferFcn  Numerator=1  Denominator=[tau_isum 1]
  R3 : TransferFcn  Numerator=1  Denominator=[tau_isum 1]
  Out1 : Outport  VectorParamsAs1DForOutWhenUnconnected=off
  wires:
  Demux11/2 -> R2/1
  R2/1 -> Mux23/2  "Pub"
  Demux11/1 -> R1/1
  Demux11/3 -> R3/1
  Mux23/1 -> Out1/1
  In1/1 -> Demux11/1
  R3/1 -> Mux23/3  "Puc"
  R1/1 -> Mux23/1  "Pua"

== system MTDC_MODEL/GRID1+MMC1/Isum_AC_Ref_Cal/DIFFERENT_REF_CALC_METHODS  ==
  v_g_pos : Inport
  Constant{1..6} (6 alike) : Constant  Value=0
  Gain1 : Gain  Gain=1/sqrt(2)
  Gain13 : Gain  Gain=1/U_ll1
  Matrix Concatenate4 : Concatenate  NumInputs=3  Mode=Multidimensional array  ConcatenateDimension=2
  Memory : Memory  InitialCondition=Vpeak_d1
  Mux11 : Mux  Inputs=3
  Mux12 : Mux  Inputs=3
  Mux5 : Mux  Inputs=3
  inv mat2 : MATLAB Function  TreatAsAtomicUnit=on
  Initial Approach : Outport  VectorParamsAs1DForOutWhenUnconnected=off
  wires:
  Mux5/1 -> Matrix Concatenate4/3
  Mux11/1 -> Matrix Concatenate4/1
  Constant5/1 -> Mux11/2
  Matrix Concatenate4/1 -> inv mat2/1(u)  "Isum_neg; -Isum_neg;  Isum_pos"
  Constant4/1 -> Mux12/1
  [v_g_pos_rms_pu] -> Mux11/1
  [v_g_pos_rms_pu] -> Mux12/2
  Constant3/1 -> Mux5/2
  [v_g_pos_rms_pu] -> Mux5/3
  inv mat2/1(y) -> Initial Approach/1
  Mux12/1 -> Matrix Concatenate4/2
  Gain1/1 -> [v_g_pos_rms_pu]
  v_g_pos/1 -> Memory/1
  Gain13/1 -> Gain1/1
  Constant1/1 -> Mux11/3
  Constant2/1 -> Mux12/3
  Constant6/1 -> Mux5/1
  Memory/1 -> Gain13/1

== system MTDC_MODEL/GRID1+MMC1/Isum_AC_Ref_Cal/Rotation4 ==
  angle : Inport
  Gain1 : Gain
  Gain2 : Gain  Gain=-1
  Gain9 : Gain  Gain=-1
  Matrix Concatenate1 : Concatenate  Mode=Multidimensional array  ConcatenateDimension=2
  Matrix Concatenate2 : Concatenate  Mode=Multidimensional array  ConcatenateDimension=2
  Mux{1..2,8..9} (4 alike) : Mux  Inputs=2
  Trigonometric Function{1,3..4,6} (4 alike) : Trigonometry  Operator=cos
  Trigonometric Function{2,5,7..8} (4 alike) : Trigonometry
  iR : Outport  VectorParamsAs1DForOutWhenUnconnected=off
  R : Outport  Port=2  VectorParamsAs1DForOutWhenUnconnected=off
  wires:
  Gain2/1 -> Mux2/1
  Matrix Concatenate2/1 -> R/1
  Gain1/1 -> Mux1/2
  Mux2/1 -> Matrix Concatenate2/2
  Mux1/1 -> Matrix Concatenate2/1
  Trigonometric Function8/1 -> Gain2/1
  Trigonometric Function2/1 -> Gain1/1
  Trigonometric Function3/1 -> Mux2/2
  Trigonometric Function1/1 -> Mux1/1
  Matrix Concatenate1/1 -> iR/1
  Gain9/1 -> Mux8/2
  angle/1 -> Trigonometric Function1/1, Trigonometric Function2/1, Trigonometric Function8/1, Trigonometric Function3/1, Trigonometric Function4/1, Trigonometric Function5/1, Trigonometric Function7/1, Trigonometric Function6/1
  Mux9/1 -> Matrix Concatenate1/2
  Mux8/1 -> Matrix Concatenate1/1
  Trigonometric Function7/1 -> Mux9/1
  Trigonometric Function5/1 -> Gain9/1
  Trigonometric Function6/1 -> Mux9/2
  Trigonometric Function4/1 -> Mux8/1

== system MTDC_MODEL/GRID1+MMC1/vsum Calculation/PR Controller1 ==
  e : Inport
  PID Controller2 : pid_lib/PID Controller  Controller=PI  Form=Parallel  TimeDomain=Continuous-time  UseExternalTs=off  SampleTime=1  IntegratorMethod=Forward Euler  FilterMethod=Forward Euler  ControllerParametersSource=internal  P=Kp_sum  I=Ki_sum  D=0  UseFilter=on  N=100  TunerSelectOption=Transfer Function Based (PID Tuner App)  InitialConditionSource=internal  InitialConditionForIntegrator=0  InitialConditionForFilter=0  DifferentiatorICPrevScaledInput=0  ExternalReset=none  TrackingMode=off  Kt=1  LimitOutput=off  SatLimitsSource=internal  UpperSaturationLimit=inf  LowerSaturationLimit=-inf  LinearizeAsGain=on  AntiWindupMode=none  Kb=1  POutMin=[]  POutMax=[]  IOutMin=[]  IOutMax=[]  DOutMin=[]  DOutMax=[]  NOutMin=[]  NOutMax=[]  SumOutMin=[]  SumOutMax=[]  SaturationOutMin=[]  SaturationOutMax=[]  PParamMin=[]  PParamMax=[]  IParamMin=[]  IParamMax=[]  DParamMin=[]  DParamMax=[]  NParamMin=[]  NParamMax=[]  KbParamMin=[]  KbParamMax=[]  KtParamMin=[]  KtParamMax=[]  KbOutMin=[]  KbOutMax=[]  KtOutMin=[]  KtOutMax=[]  IntegratorOutMin=[]  IntegratorOutMax=[]  FilterOutMin=[]  FilterOutMax=[]  SumI1OutMin=[]  SumI1OutMax=[]  SumI2OutMin=[]  SumI2OutMax=[]  SumI3OutMin=[]  SumI3OutMax=[]  SumI4OutMin=[]  SumI4OutMax=[]  SumDOutMin=[]  SumDOutMax=[]  DifferentiatorOutMin=[]  DifferentiatorOutMax=[]  FilterDiffOutCoefMin=[]  FilterDiffOutCoefMax=[]  ReciprocalOutMin=[]  ReciprocalOutMax=[]  SumDenOutMin=[]  SumDenOutMax=[]  SumNumOutMin=[]  SumNumOutMax=[]  DivideOutMin=[]  DivideOutMax=[]  UdiffTsProdOutMin=[]  UdiffTsProdOutMax=[]  NTsProdOutMin=[]  NTsProdOutMax=[]  UintegralTsProdOutMin=[]  UintegralTsProdOutMax=[]  UngainTsProdOutMin=[]  UngainTsProdOutMax=[]  IntegratorContinuousStateAttributes=''  IntegratorStateMustResolveToSignalObject=off  IntegratorRTWStateStorageClass=Auto  FilterContinuousStateAttributes=''  FilterStateMustResolveToSignalObject=off  FilterRTWStateStorageClass=Auto  ParallelPVariant=InternalParameters  IdealPVariant=Disabled  IVariant=InternalParameters  DVariant=Disabled  IntegratorVariant=Continuous  SatVariant=Disabled  AWVariant=Passthrough  PCopyVariant=Disabled  TRVariant=Disabled  FdbkBlocksVariant=Forward  IdealPFdbkVariant=Disabled  SatFdbkVariant=Disabled  DerivativeFilterVariant=Disabled  NVariant=Disabled  NCopyVariant=Disabled_SignalSpec  FilterICVariant=Disabled  IntegratorICVariant=InternalICs  ExternalResetVariant=Disabled  TRSumVariant=Passthrough  SumFdbkVariant=Disabled  SumVariant=Sum_PI  TsampFilterVariant=InternalTs  TsampNgainVariant=Passthrough  TsampIntegralVariant=Passthrough  ExternalSaturationOutDataTypeStr=Inherit: Same as second input
  Sum1 : Sum  Inputs=++|
  Transfer Fcn : TransferFcn  Numerator=PR.num{1}  Denominator=PR.den{1}
  v : Outport
  wires:
  e/1 -> Transfer Fcn/1, PID Controller2/1
  Transfer Fcn/1 -> Sum1/2
  Sum1/1 -> v/1
  PID Controller2/1 -> Sum1/1

== system MTDC_MODEL/GRID1+MMC1/vsum Calculation/PR Controller2 ==
  e : Inport
  PID Controller2 : pid_lib/PID Controller  Controller=PI  Form=Parallel  TimeDomain=Continuous-time  UseExternalTs=off  SampleTime=1  IntegratorMethod=Forward Euler  FilterMethod=Forward Euler  ControllerParametersSource=internal  P=Kp_sum  I=Ki_sum  D=0  UseFilter=on  N=100  TunerSelectOption=Transfer Function Based (PID Tuner App)  InitialConditionSource=internal  InitialConditionForIntegrator=0  InitialConditionForFilter=0  DifferentiatorICPrevScaledInput=0  ExternalReset=none  TrackingMode=off  Kt=1  LimitOutput=off  SatLimitsSource=internal  UpperSaturationLimit=inf  LowerSaturationLimit=-inf  LinearizeAsGain=on  AntiWindupMode=none  Kb=1  POutMin=[]  POutMax=[]  IOutMin=[]  IOutMax=[]  DOutMin=[]  DOutMax=[]  NOutMin=[]  NOutMax=[]  SumOutMin=[]  SumOutMax=[]  SaturationOutMin=[]  SaturationOutMax=[]  PParamMin=[]  PParamMax=[]  IParamMin=[]  IParamMax=[]  DParamMin=[]  DParamMax=[]  NParamMin=[]  NParamMax=[]  KbParamMin=[]  KbParamMax=[]  KtParamMin=[]  KtParamMax=[]  KbOutMin=[]  KbOutMax=[]  KtOutMin=[]  KtOutMax=[]  IntegratorOutMin=[]  IntegratorOutMax=[]  FilterOutMin=[]  FilterOutMax=[]  SumI1OutMin=[]  SumI1OutMax=[]  SumI2OutMin=[]  SumI2OutMax=[]  SumI3OutMin=[]  SumI3OutMax=[]  SumI4OutMin=[]  SumI4OutMax=[]  SumDOutMin=[]  SumDOutMax=[]  DifferentiatorOutMin=[]  DifferentiatorOutMax=[]  FilterDiffOutCoefMin=[]  FilterDiffOutCoefMax=[]  ReciprocalOutMin=[]  ReciprocalOutMax=[]  SumDenOutMin=[]  SumDenOutMax=[]  SumNumOutMin=[]  SumNumOutMax=[]  DivideOutMin=[]  DivideOutMax=[]  UdiffTsProdOutMin=[]  UdiffTsProdOutMax=[]  NTsProdOutMin=[]  NTsProdOutMax=[]  UintegralTsProdOutMin=[]  UintegralTsProdOutMax=[]  UngainTsProdOutMin=[]  UngainTsProdOutMax=[]  IntegratorContinuousStateAttributes=''  IntegratorStateMustResolveToSignalObject=off  IntegratorRTWStateStorageClass=Auto  FilterContinuousStateAttributes=''  FilterStateMustResolveToSignalObject=off  FilterRTWStateStorageClass=Auto  ParallelPVariant=InternalParameters  IdealPVariant=Disabled  IVariant=InternalParameters  DVariant=Disabled  IntegratorVariant=Continuous  SatVariant=Disabled  AWVariant=Passthrough  PCopyVariant=Disabled  TRVariant=Disabled  FdbkBlocksVariant=Forward  IdealPFdbkVariant=Disabled  SatFdbkVariant=Disabled  DerivativeFilterVariant=Disabled  NVariant=Disabled  NCopyVariant=Disabled_SignalSpec  FilterICVariant=Disabled  IntegratorICVariant=InternalICs  ExternalResetVariant=Disabled  TRSumVariant=Passthrough  SumFdbkVariant=Disabled  SumVariant=Sum_PI  TsampFilterVariant=InternalTs  TsampNgainVariant=Passthrough  TsampIntegralVariant=Passthrough  ExternalSaturationOutDataTypeStr=Inherit: Same as second input
  Sum1 : Sum  Inputs=++|
  Transfer Fcn : TransferFcn  Numerator=PR.num{1}  Denominator=PR.den{1}
  v : Outport
  wires:
  PID Controller2/1 -> Sum1/1
  Sum1/1 -> v/1
  Transfer Fcn/1 -> Sum1/2
  e/1 -> PID Controller2/1, Transfer Fcn/1

== system MTDC_MODEL/GRID1+MMC1/vsum Calculation/PR Controller3 ==
  e : Inport
  PID Controller2 : pid_lib/PID Controller  Controller=PI  Form=Parallel  TimeDomain=Continuous-time  UseExternalTs=off  SampleTime=1  IntegratorMethod=Forward Euler  FilterMethod=Forward Euler  ControllerParametersSource=internal  P=Kp_sum  I=Ki_sum  D=0  UseFilter=on  N=100  TunerSelectOption=Transfer Function Based (PID Tuner App)  InitialConditionSource=internal  InitialConditionForIntegrator=0  InitialConditionForFilter=0  DifferentiatorICPrevScaledInput=0  ExternalReset=none  TrackingMode=off  Kt=1  LimitOutput=off  SatLimitsSource=internal  UpperSaturationLimit=inf  LowerSaturationLimit=-inf  LinearizeAsGain=on  AntiWindupMode=none  Kb=1  POutMin=[]  POutMax=[]  IOutMin=[]  IOutMax=[]  DOutMin=[]  DOutMax=[]  NOutMin=[]  NOutMax=[]  SumOutMin=[]  SumOutMax=[]  SaturationOutMin=[]  SaturationOutMax=[]  PParamMin=[]  PParamMax=[]  IParamMin=[]  IParamMax=[]  DParamMin=[]  DParamMax=[]  NParamMin=[]  NParamMax=[]  KbParamMin=[]  KbParamMax=[]  KtParamMin=[]  KtParamMax=[]  KbOutMin=[]  KbOutMax=[]  KtOutMin=[]  KtOutMax=[]  IntegratorOutMin=[]  IntegratorOutMax=[]  FilterOutMin=[]  FilterOutMax=[]  SumI1OutMin=[]  SumI1OutMax=[]  SumI2OutMin=[]  SumI2OutMax=[]  SumI3OutMin=[]  SumI3OutMax=[]  SumI4OutMin=[]  SumI4OutMax=[]  SumDOutMin=[]  SumDOutMax=[]  DifferentiatorOutMin=[]  DifferentiatorOutMax=[]  FilterDiffOutCoefMin=[]  FilterDiffOutCoefMax=[]  ReciprocalOutMin=[]  ReciprocalOutMax=[]  SumDenOutMin=[]  SumDenOutMax=[]  SumNumOutMin=[]  SumNumOutMax=[]  DivideOutMin=[]  DivideOutMax=[]  UdiffTsProdOutMin=[]  UdiffTsProdOutMax=[]  NTsProdOutMin=[]  NTsProdOutMax=[]  UintegralTsProdOutMin=[]  UintegralTsProdOutMax=[]  UngainTsProdOutMin=[]  UngainTsProdOutMax=[]  IntegratorContinuousStateAttributes=''  IntegratorStateMustResolveToSignalObject=off  IntegratorRTWStateStorageClass=Auto  FilterContinuousStateAttributes=''  FilterStateMustResolveToSignalObject=off  FilterRTWStateStorageClass=Auto  ParallelPVariant=InternalParameters  IdealPVariant=Disabled  IVariant=InternalParameters  DVariant=Disabled  IntegratorVariant=Continuous  SatVariant=Disabled  AWVariant=Passthrough  PCopyVariant=Disabled  TRVariant=Disabled  FdbkBlocksVariant=Forward  IdealPFdbkVariant=Disabled  SatFdbkVariant=Disabled  DerivativeFilterVariant=Disabled  NVariant=Disabled  NCopyVariant=Disabled_SignalSpec  FilterICVariant=Disabled  IntegratorICVariant=InternalICs  ExternalResetVariant=Disabled  TRSumVariant=Passthrough  SumFdbkVariant=Disabled  SumVariant=Sum_PI  TsampFilterVariant=InternalTs  TsampNgainVariant=Passthrough  TsampIntegralVariant=Passthrough  ExternalSaturationOutDataTypeStr=Inherit: Same as second input
  Sum1 : Sum  Inputs=++|
  Transfer Fcn : TransferFcn  Numerator=PR.num{1}  Denominator=PR.den{1}
  v : Outport
  wires:
  e/1 -> Transfer Fcn/1, PID Controller2/1
  Transfer Fcn/1 -> Sum1/2
  Sum1/1 -> v/1
  PID Controller2/1 -> Sum1/1

== system MTDC_MODEL/GRID2+MMC2/Current loop1/1SMC ==
  iq : Inport
  Ref_iq : Inport  Port=2
  Ref_id : Inport  Port=3
  id : Inport  Port=4
  Add : Sum  Inputs=---
  Gain2 : Gain  Gain=(Rg_1+Ra_1/2)
  Gain3 : Gain  Gain=Kq
  Gain4 : Gain  Gain=Qq
  Gain5 : Gain  Gain=(Lg_1+La_1/2)
  Gain6 : Gain  Gain=(Lg_1+La_1/2)*2*pi*50
  Scope : Scope  NumInputPorts=2
  Sign : Signum  ZeroCross=off
  Sum2 : Sum  Inputs=|++
  Sum5 : Sum  Inputs=|+-
  Out1 : Outport
  Sq : Outport  Port=2
  wires:
  Ref_id/1 -> Gain6/1
  Sum5/1 -> Sign/1, Sq/1, Gain3/1  "Sq"
  iq/1 -> Sum5/2
  Add/1 -> Scope/1, Out1/1
  Gain6/1 -> Add/1
  Gain2/1 -> Add/2
  Ref_iq/1 -> Sum5/1, Gain2/1
  Sum2/1 -> Gain5/1
  Gain4/1 -> Sum2/1
  Gain3/1 -> Sum2/2
  Sign/1 -> Gain4/1
  Gain5/1 -> Add/3, Scope/2

== system MTDC_MODEL/GRID2+MMC2/Current loop1/PLCS ==
  iq : Inport
  Ref_iq : Inport  Port=2
  Ref_id : Inport  Port=3
  id : Inport  Port=4
  Abs2 : Abs
  Add : Sum  Inputs=---
  Add1 : Sum
  Derivative : Derivative
  Gain1 : Gain  Gain=20000
  Gain14 : Gain  Gain=3900
  Gain2 : Gain  Gain=(Rg_1+Ra_1/2)
  Gain3 : Gain  Gain=(Lg_1+La_1/2)
  Gain6 : Gain  Gain=(Lg_1+La_1/2)*2*pi*50
  Product : Product
  Scope : Scope  NumInputPorts=2
  Sign1 : Signum
  Sign2 : Signum
  Sqrt3 : Sqrt  SaturateOnIntegerOverflow=on
  Sum5 : Sum  Inputs=|+-
  Out1 : Outport
  Sq : Outport  Port=2
  wires:
  Ref_id/1 -> Gain6/1
  Sum5/1 -> Sign1/1, Scope/2, Sq/1, Derivative/1, Abs2/1  "Sq"
  iq/1 -> Sum5/2
  Add/1 -> Out1/1
  Gain6/1 -> Add/1
  Gain2/1 -> Add/2
  Ref_iq/1 -> Gain2/1, Sum5/1
  Gain3/1 -> Scope/1, Add/3
  Abs2/1 -> Sqrt3/1
  Sign1/1 -> Product/1
  Sqrt3/1 -> Product/2
  Product/1 -> Gain14/1
  Gain14/1 -> Add1/1
  Derivative/1 -> Add1/2
  Add1/1 -> Sign2/1
  Gain1/1 -> Gain3/1
  Sign2/1 -> Gain1/1

== system MTDC_MODEL/GRID2+MMC2/Current loop1/SMC-Dynamic ==
  iq : Inport
  Ref_iq : Inport  Port=2
  Ref_id : Inport  Port=3
  vzq : Inport  Port=4
  Add : Sum
  Add2 : Sum  Inputs=---
  Derivative2 : Derivative
  Gain1 : Gain  Gain=0.002
  Gain2 : Gain  Gain=(Rg_1+Ra_1/2)
  Gain3 : Gain  Gain=0.02
  Gain4 : Gain  Gain=0.00416
  Gain6 : Gain  Gain=(Lg_1+La_1/2)*2*pi*50
  Integrator1 : Integrator
  Integrator2 : Integrator
  Scope : Scope  NumInputPorts=3
  Sign : Signum  ZeroCross=off
  Sum5 : Sum  Inputs=|+-
  To File : ToFile  Filename=iq_ref.mat  MatrixName=ans99  SaveFormat=Timeseries
  To File1 : ToFile  Filename=iq.mat  MatrixName=ans100  SaveFormat=Timeseries
  Out1 : Outport
  Sq : Outport  Port=2
  wires:
  Ref_id/1 -> Gain6/1
  Sum5/1 -> Integrator1/1, Sign/1, Sq/1  "Sq"
  iq/1 -> To File1/1, Sum5/2
  Ref_iq/1 -> To File/1, Sum5/1, Gain2/1
  Sign/1 -> Gain3/1
  Integrator1/1 -> Gain1/1
  Gain6/1 -> Add2/1
  Gain2/1 -> Add2/2
  Gain1/1 -> Add/2
  Add/1 -> Gain4/1
  Gain4/1 -> Add2/3
  Add2/1 -> Out1/1
  Gain3/1 -> Integrator2/1
  Integrator2/1 -> Add/1

== system MTDC_MODEL/GRID2+MMC2/Current loop1/SMC1 ==
  id : Inport
  Ref_id : Inport  Port=2
  Ref_iq : Inport  Port=3
  iq : Inport  Port=4
  Add : Sum  Inputs=+--
  Gain2 : Gain  Gain=(Rg_1+Ra_1/2)
  Gain3 : Gain  Gain=Kd*0.7
  Gain4 : Gain  Gain=Qd
  Gain5 : Gain  Gain=(Lg_1+La_1/2)
  Gain6 : Gain  Gain=(Lg_1+La_1/2)*2*pi*50
  Sign : Signum  ZeroCross=off
  Sum2 : Sum  Inputs=|++
  Sum5 : Sum  Inputs=|+-
  Out1 : Outport
  Sd : Outport  Port=2
  wires:
  Sum2/1 -> Gain5/1
  Gain4/1 -> Sum2/1
  Gain3/1 -> Sum2/2
  Sign/1 -> Gain4/1
  Ref_id/1 -> Gain2/1, Sum5/1
  Gain6/1 -> Add/1
  Gain2/1 -> Add/2
  Gain5/1 -> Add/3
  id/1 -> Sum5/2
  Sum5/1 -> Gain3/1, Sd/1, Sign/1  "Sd"
  Add/1 -> Out1/1
  Ref_iq/1 -> Gain6/1

== system MTDC_MODEL/GRID2+MMC2/Current loop1/ST-SMC ==
  iq : Inport
  Ref_iq : Inport  Port=2
  Ref_id : Inport  Port=3
  id : Inport  Port=4
  Abs2 : Abs
  Add : Sum  Inputs=---
  Add1 : Sum
  Gain14 : Gain  Gain=4000
  Gain17 : Gain  Gain=4000
  Gain2 : Gain  Gain=(Rg_1+Ra_1/2)
  Gain5 : Gain  Gain=(Lg_1+La_1/2)
  Gain6 : Gain  Gain=(Lg_1+La_1/2)*2*pi*50
  Integrator2 : Integrator
  Product2 : Product
  Scope : Scope  NumInputPorts=2
  Sign2 : Signum
  Sqrt3 : Sqrt  SaturateOnIntegerOverflow=on
  Sum5 : Sum  Inputs=|+-
  Out1 : Outport
  Sq : Outport  Port=2
  wires:
  Gain5/1 -> Scope/2, Add/3
  Ref_iq/1 -> Sum5/1, Gain2/1
  Gain2/1 -> Add/2
  Gain6/1 -> Add/1
  Add/1 -> Scope/1, Out1/1
  iq/1 -> Sum5/2
  Sum5/1 -> Sq/1, Abs2/1, Sign2/1  "Sq"
  Ref_id/1 -> Gain6/1
  Sign2/1 -> Integrator2/1, Product2/1
  Product2/1 -> Gain14/1
  Sqrt3/1 -> Product2/2
  Abs2/1 -> Sqrt3/1
  Integrator2/1 -> Gain17/1
  Add1/1 -> Gain5/1
  Gain17/1 -> Add1/1
  Gain14/1 -> Add1/2
